simulink library "CampusEnergyModeling"  (Simulink 8.1)
settings: Solver=ode45  StartTime=0.0  StopTime=10.0  RelTol=1e-3
values from neighbouring files (symbols this model uses):
  a = alpha    [GenericInverter_cb.m]
  b = beta    [GenericInverter_cb.m]
  c = gamma    [GenericInverter_cb.m]
  look_Pin = lookup_out ./ lookup_eff    [GenericInverter_cb.m]
  look_Pout = lookup_out    [GenericInverter_cb.m]
undefined symbols (not defined in the file or in its folder): j, magnitude
libraries: powerlib x5, simulink x3
settings Model: Creator=sfrank1  LastModifiedBy=sfrank1

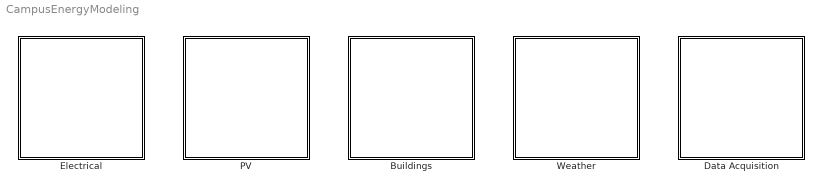
== system CampusEnergyModeling ==
  Buildings : Subsystem  Tag=Weather  Description=Contains blocks for acquiring and manipulating weather data.
      mask Display: disp('Buildings')
  Data Acquisition : Subsystem  Tag=Weather  Description=Contains blocks for acquiring and manipulating weather data.
      mask Display: disp('Data\nAcquisition')
  Electrical : Subsystem  Tag=Weather  Description=Contains blocks for acquiring and manipulating weather data.
      mask Display: disp('Electrical')
  PV : Subsystem  Tag=Weather  Description=Contains blocks for acquiring and manipulating weather data.
      mask Display: disp('PV')
  Weather : Subsystem  Tag=Weather  Description=Contains blocks for acquiring and manipulating weather data.
      mask Display: disp('Weather')

== system CampusEnergyModeling/Buildings ==
  E+ Building : M-S-Function  FunctionName=mlepSimulinkBlk  Parameters=progname, modelfile, weatherfile, workdir, timeout, port, host, bcvtbdir, deltaT, noutputd  mask(EnergyPlus Cosimulation){progname='C:\EnergyPlusV8-0-0\RunEPlus.bat', modelfile='\path\to\dir\idf_file', weatherfile='USA_IL_Chicago-OHare.Intl.AP.725300_TMY3', workdir='\path\to\dir', timeout=80000, port=0, host='', bcvtbdir='', deltaT=900, noutputd=2}
      mask prompts: progname "E+ Executable Path"; modelfile "IDF File (without extension)"; weatherfile "Weather Profile"; workdir "Working Directory"; timeout "Timeout (in milliseconds)"; port "Socket Port (0 = any available)"; host "Socket Host ('' = local host)"; bcvtbdir "BCVTB Directory"; deltaT "Time Step (in seconds)"; noutputd "Number of Real Outputs"
      mask help: This block implements cosimulation with EnergyPlus by allowing Simulink to exchange input and output data with it. Currently, EnergyPlus only supports real data.
      mask Help:
      | This block implements cosimulation with EnergyPlus by allowing Simulink to exchange input and output data with it.
      | 
      | When a simulation starts, EnergyPlus is also started. It will then run in parallel with Simulink. They exchange input and output data via socket communication. When the simulation terminates, EnergyPlus will exit.
      | 
      | Refer to the manuals of MLE+ and/or BCVTB/EnergyPlus for details.
      | 
      | INPUTS:
      | - real: real vector input to EnergyPlus.
      | 
      | OUTPUTS:
      | - flag: status of EnergyPlus (0 if OK, if flag is non-zero, the simulation should stop).
      | - time: current simulation time of EnergyPlus, in seconds.
      | - real: real vector output from EnergyPlus.
      mask Display:
      | image(imread('building.png'))
      | disp('E+\nCosimulation');
      | 
      | % Inputs
      | port_label('input', 1, 'real');
      | 
      | % Outputs
      | port_label('output', 1, 'flag');
      | port_label('output', 2, 'time');
      | port_label('output', 3, 'real');
  E+ Plant : M-S-Function  FunctionName=mlepSimulinkBlk  Parameters=progname, modelfile, weatherfile, workdir, timeout, port, host, bcvtbdir, deltaT, noutputd  mask(EnergyPlus Cosimulation){progname='C:\EnergyPlusV8-0-0\RunEPlus.bat', modelfile='\path\to\dir\idf_file', weatherfile='USA_IL_Chicago-OHare.Intl.AP.725300_TMY3', workdir='\path\to\dir', timeout=80000, port=0, host='', bcvtbdir='', deltaT=900, noutputd=2}
      mask prompts: progname "E+ Executable Path"; modelfile "IDF File (without extension)"; weatherfile "Weather Profile"; workdir "Working Directory"; timeout "Timeout (in milliseconds)"; port "Socket Port (0 = any available)"; host "Socket Host ('' = local host)"; bcvtbdir "BCVTB Directory"; deltaT "Time Step (in seconds)"; noutputd "Number of Real Outputs"
      mask help: This block implements cosimulation with EnergyPlus by allowing Simulink to exchange input and output data with it. Currently, EnergyPlus only supports real data.
      mask Help:
      | This block implements cosimulation with EnergyPlus by allowing Simulink to exchange input and output data with it.
      | 
      | When a simulation starts, EnergyPlus is also started. It will then run in parallel with Simulink. They exchange input and output data via socket communication. When the simulation terminates, EnergyPlus will exit.
      | 
      | Refer to the manuals of MLE+ and/or BCVTB/EnergyPlus for details.
      | 
      | INPUTS:
      | - real: real vector input to EnergyPlus.
      | 
      | OUTPUTS:
      | - flag: status of EnergyPlus (0 if OK, if flag is non-zero, the simulation should stop).
      | - time: current simulation time of EnergyPlus, in seconds.
      | - real: real vector output from EnergyPlus.
      mask Display:
      | image(imread('chiller_plant.jpg'))
      | disp('E+\nCosimulation');
      | 
      | % Inputs
      | port_label('input', 1, 'real');
      | 
      | % Outputs
      | port_label('output', 1, 'flag');
      | port_label('output', 2, 'time');
      | port_label('output', 3, 'real');

== system CampusEnergyModeling/Data Acquisition ==

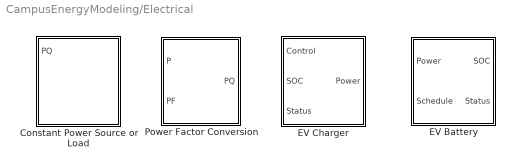
== system CampusEnergyModeling/Electrical ==
  Constant Power Source or Load : Subsystem  mask(Constant Power Source/Load){Conven=source, PNom=5000, QNom=2000, VNom=480, fNom=60, VLow=0.7}
      mask prompts: Conven "Electrical convention"; PNom "Nominal three-phase real power (W)"; QNom "Nominal three-phase reactive power (VAR)"; VNom "Nominal line-to-line voltage (VRMS)"; fNom "Nominal frequency (Hz)"; VLow "Lower voltage limit (pu)"
      mask help: Implements a controllable three-phase, constant power source or load, where VI* = P + jQ (in per-unit).
      mask init:
      | % Call initialization to calculate block variables
      | InputGain = ...
      |     ConstantPowerSourceLoad_cb(gcb, 'init', ...
      |     Conven, PNom, QNom, VNom, fNom, VLow);
      mask Help:
      | Implements a controllable three-phase, constant power source or load in SimPowerSystems (phasor mode). The load characteristic is given by P + jQ = sqrt(3)VI*, in which
      |     V = Positive sequence line-to-line voltage (V)
      |     I = Positive sequence phase current (A)
      |     P = Positive sequence real power (from PQ input)
      |     Q = Positive sequence reactive power (from PQ input)
      | 
      | The block supplies P + jQ if the source convention is specified and consumes P + jQ if the load convention is specified.
      | 
      | The nominal input fields in the mask are used to initialize the block parameters. If the nominal values are close to the actual values during simulation, then the block will converge more rapidly.
      | 
      | If the positive sequence voltage falls below the per-unit lower voltage limit (on the base specified by the nominal line-to-line voltage), then the block will behave as a constant current source rather than a constant power source, with the current magnitude capped at the level required to supply full power at V = 0.7 pu. This feature avoids current runaway that would otherwise occur during voltage collapes.
      | 
      | NOTE: This block is compatible only with SimPowerSystems' phasor simulation mode.
      mask TypeOptions Conven: source | load
  EV Battery : Subsystem  mask(Electric Vehicle Battery){capacity=24000, initSOC=0.3}
      mask prompts: capacity "Battery capacity (Wh)"; initSOC "Initial state of charge (fraction)"
      mask help: Implements a simple, lossless model for an electric vehicle (EV) battery.
      mask Help:
      | Implements a simple, lossless model for an electric vehicle (EV) battery.
      | 
      | The block accepts the following inputs:
      | •	Power = The charging power for the battery (W)
      | •	Schedule = 1 if the EV is connected to the charging station, 0 otherwise
      | 
      | The block outputs two signals:
      | •	SOC = The battery state of charge (fraction)
      | •	Status = EV status: -1 for not present, 0 for present and accepting charge, 1 for present but battery full
      | 
      | Internally, the battery is modeled using a simple integrator for the input power, capped at 100% SOC. Battery SOC resets to the specified initial value whenever the EV first connects to the charging station. The battery is lossless.
  EV Charger : Subsystem  mask(Electric Vehicle Charging Station){rating=6240, capacity=24000, maxresponse=1000, ramp=1000}
      mask prompts: rating "Charger rating (W)"; capacity "Connected EV battery capacity (Wh)"; maxresponse "Desired +/- regulatory response capability (W)"; ramp "Maximum ramp rate (W/s)"
      mask help: Implements a simple model for an electric vehicle charging station. Accepts connections for the EV state of charge and status as well as an external control signal requesting a regulatory deviation from the current charging setpoint. Outputs a charging power.
      mask Help:
      | Implements a simple model for an electric vehicle (EV) charging station.
      | 
      | The block accepts the following inputs:
      | •	Control = Signal requesting regulatory control of power consumed (+/- deviation from setpoint) (W)
      | •	SOC = EV battery state of charge (fraction)
      | •	Status = EV status: -1 for not present, 0 for present and accepting charge, 1 for present but battery full
      | 
      | The block outputs the charging power to the EV battery.
      | 
      | The charger uses a preset charging power profile based on the EV battery state of charge (SOC). As the SOC approaches 100%, the charger tapers the charge rate to zero. In addition, the charger monitors the connection status of the EV and sets charging power to zero if the EV is disconnected or has a full battery.
      | 
      | The 'Control' signal requests regulatory control of the EV charging load as a deviation from the current charging setpoint. This allows the EV charger to participate in demand response or regulation of distributed generation (such as smoothing output from a photovoltaic array). The charger attempts to maintain the active response capability specified in the block mask by operating at less than maximum charging capacity. It can then respond to the control signal within its present charging limits.
      | 
      | For example, if, given the current battery SOC, the charging profile for the EV battery specifies 5000 W and the requested regulatory response capability is +/- 1000 W, then the EV charger will charge at a setpoint of 4000 W +/- the requested control action, within the limits of the charger. If the requested control action is -500 W, then the EV charger will reduce output to 4000 - 500 = 3500 W.
      | 
      | The ability of the charger to respond to the control action is limited by several factors:
      | 1.	The output cannot exceed either its specified rating or the maximum charge rate given by the battery charging profile.
      | 2.	The output cannot be less than zero.
      | 3.	The output cannot change at a rate greater than the specified maximum ramp rate (W/s).
  Power Factor Conversion : Subsystem  mask(Power Factor Conversion){pfType=Lagging}
      mask prompts: pfType "Type of power factor"
      mask help: Converts a real input power and power factor to a vector of real and reactive power.
      mask init:
      | % Set multiplier for Q based on load type
      | if pfType == 1
      |     % Leading
      |     leadlag = -1;
      | else
      |     % Lagging
      |     leadlag = 1;
      | end
      mask Help: Converts a real input power and power factor to a vector of real and reactive power. The output is a vector [P Q] computed from the input power P, input power factor PF, and whether the signal indicates leading or lagging power (selectable in the block mask).
      mask TypeOptions pfType: Leading | Lagging

== system CampusEnergyModeling/PV ==
  Generic Inverter : Subsystem  mask(Generic Inverter){model_type=Fixed Efficiency, fixed_eff=0.95, alpha=1, beta=0.01, gamma=0.001, lookup_pair=Input Power + Output Power, lookup_in=[0, 10, 25, 50, 75, 100], lookup_out=[0, 9, 24, 49, 73, 97], lookup_eff=[0.10, 0.80, 0.87, 0.93, 0.90, 0.88]}
      mask prompts: model_type "Inverter model"; fixed_eff "Efficiency"; alpha "Constant loss coefficient (W)"; beta "Linear loss coefficient (W/W)"; gamma "Quadratic loss coefficient (W/W²)"; lookup_pair "Specify..."; lookup_in "Input power (W)"; lookup_out "Output power (W)"; lookup_eff "Efficiency"
      mask help:
      | Implements the efficiency characteristic for a generic PV inverter using one of three models:
      | - Fixed efficiency
      | - Quadratic loss model
      | - Lookup table
      |
      | See the help for details for each of these models.
      mask init:
      | % Call initialization to calculate block variables
      | [a, b, c, look_Pin, look_Pout] = ...
      |     GenericInverter_cb(gcb, 'init', model_type, ...
      | 	fixed_eff, alpha, beta, gamma, ...
      |     lookup_pair, lookup_in, lookup_out, lookup_eff);
      mask Help:
      | This block implements the efficiency characteristic for a generic PV inverter using one of three models:
      | - Fixed efficiency
      | - Quadratic loss model
      | - Lookup table
      | 
      | Fixed Efficiency:
      | Specify the fixed inverter efficiency as a fraction.
      | 
      | Quadratic Loss Model:
      | Specify the loss model coefficients such that
      | Pout = Pin - (alpha + beta*Pin + gamma*Pin²).
      | 
      | Lookup Table:
      | Specify two of the following three vectors: input power, output power, and efficiency. Efficiencies must be entered as fractions and vector lengths must match. The block automatically calculates the appropriate input-output power characteristic from the inputs provided according to the relationship Efficiency = Pout / Pin.
      | 
      | CAUTION: When using the lookup table, do not include zeros in the efficiency vector. Otherwise, a divide by zero error may result.
      mask TypeOptions model_type: Fixed Efficiency | Quadratic | Lookup Table
      mask Callback model_type:
      | % Dynamic mask callback
      | GenericInverter_cb(gcb, 'model_type')
      mask TypeOptions lookup_pair: Input Power + Output Power | Input Power + Efficiency | Output Power + Efficiency
      mask Callback lookup_pair:
      | % Dynamic mask callback
      | GenericInverter_cb(gcb, 'lookup_pair')
  PV Smoothing : TransferFcn  Denominator=[tau 1]  mask(Photovoltaic Array Smoothing){sel=Array Size and Power Density, tc=15, area=33000, size=1e6, density=150, coverage=0.2}
      mask prompts: sel "Specify..."; tc "Time constant (s)"; area "Array area (m²)"; size "Array size (W)"; density "Panel nominal power density (W/m²)"; coverage "Panel ground coverage ratio (fraction)"
      mask help: Implements a low pass filter to model the smoothing effect of a utility-scale PV array.
      mask init:
      | % Call initialization to calculate block variables
      | tau = PVSmoothing_cb(gcb, 'init', ...
      |     sel, tc, area, size, density, coverage);
      mask Help:
      | This block implements a low pass filter to model the smoothing effect of a utility-scale PV array per the empirical model presented in Marcos et al. (2011) (see References). The smoothing is done by a unity-gain low pass filter with transfer function
      | 
      | Output / Input = 1 / (tau*s + 1)
      | 
      | in which time constant tau may either be defined directly or estimated from the array area. The empirical formula of Marcos et al. estimates tau as
      | 
      | tau = sqrt(A) / (2*pi*0.020)
      | 
      | in which A is the physical array area in hectares (1 Ha = 10000 m²). Array area A may be specified directly or calculated from the array size, panel power density, and ground coverage ratio (defined as the fraction of ground area occupied by the actual PV panels).
      | 
      | Notes:
      | 1. This block includes a continuous time low pass filter. Use caution when attempting to use this block within models with fixed time larger than the smoothing time constant; the Simulink solver may generate an error.
      | 
      | References:
      | J. Marcos et al., "From irradiance to output power fluctuations: the PV plant as a low pass filter", Progress In Photovoltaics: Research And Applications, 2011, 19, 505-510.
      mask TypeOptions sel: Time Constant | Array Area | Array Size and Power Density
      mask Callback sel: PVSmoothing_cb(gcb, 'dynamic_mask')
      mask Display: plot([1 2 3],[1 1 0])
  PVWatts Cosimulation : M-S-Function  FunctionName=pvwatts_sfun  Parameters=lat, lon, start_time, tz, time_step, system_size, derate, azimuth, tilt, track_mode, rotlim, t_ref, t_noct, gamma, i_ref, poa_cutin, init_tcell, init_poa, output_dc, output_celltemp, output_poa  mask(PVWatts Cosimulation){lat=39.74, lon=-105.18, start_time=2012-01-01 00:00:00, tz=-6, time_step=600, system_size=1000, derate=0.95, azimuth=180, tilt=39.74, use_lat_tilt=on, track_mode=Fixed, rotlim=45, use_cell_data=off, t_ref=25, t_noct=45, gamma=-0.5, i_ref=1000, poa_cutin=0, init_tcell=25, init_poa=0, output_dc=on, output_celltemp=on, output_poa=on}
      mask prompts: lat "Latitude"; lon "Longitude"; start_time "Initial date/time (yyyy-mm-dd HH:MM:SS)"; tz "Time zone (offset from UTC)"; time_step "Time step (s)"; system_size "Array nameplate capacity (W)"; derate "System derate factor (0-1)"; azimuth "Azimuth angle (N = 0°, E = 90°, S = 180°, W = 270°)"; tilt "Tilt angle"; use_lat_tilt "Use latitude tilt"; track_mode "Tracking mode"; rotlim "Tracker rotation limit (+/-)"; use_cell_data "Customize photovoltaic cell data"; t_ref "Reference cell temperature (°C)"; t_noct "Nominal operating cell temperature (°C)"; gamma "Maximum power temperature coefficient (%/°C)"; i_ref "Irradiance condition for cell rating (W/m²)"; poa_cutin "Minimum irradiance for operation (W/m²)"; init_tcell "Initial cell temperature (°C)"; init_poa "Initial plane of array irradiance (W/m²)"; output_dc "Output DC power (W)"; output_celltemp "Output cell temperature (°C)"; output_poa "Output plane of array irradiance (W/m²)"
      mask help:
      | This block implements cosimulation of a photovoltaic (PV) array using the PVWatts module of the SAM Simulation Code (SSC) SDK. Data entry is organized in four tabs:
      | 1. Time and Location: where the array is located and when the simulation occurs.
      | 2. Array: PV array nameplate rating and physical characteristics.
      | 3. Cell: Customized model parameters for the PV cells (optional).
      | 4. Simulation: Initial conditions and simulation options.
      |
      | See the block help for more information.
      mask init:
      | PVWatts_cb(gcb, 'redraw_mask');
      mask Help:
      | This block implements cosimulation of a photovoltaic (PV) array using the PVWatts (pvwattsfunc) module of the SAM Simulation Code (SSC) SDK. The cosimulation runs in SSC at the time step specified in the 'Time and Location' tab (which need not be identical to the Simulink time step).
      | 
      | The block inputs accept weather data synced to the simulation time stamp:
      | 1. Beam irradiance (W/m²) - Also known as "direct normal irradiance"
      | 2. Diffuse irradiance (W/m²) - Also known as "diffuse horizontal irradiance"
      | 3. Ambient temperature (°C)
      | 4. Wind speed (m/s)
      | 
      | The block mask provides inputs for most (although not all) of the remaining PV array model parameters available for PVWatts in SSC, such as the array ratings, physical location and orientation, PV cell characteristics, etc. The four input tabs in the block mask are:
      | 1. Time and Location: where the array is located and when the simulation occurs.
      | 2. Array: PV array nameplate rating and physical characteristics.
      | 3. Cell: Customized model parameters for the PV cells (optional).
      | 4. Simulation: Initial conditions and simulation options.
      | 
      | The block outputs are, in order:
      | 1. Array DC output power (W)
      | 2. Array cell temperature (°C)
      | 3. Plane of array irradiance (W/m²)
      | Each output may be individually enabled or disabled on the 'Simulation' tab. Please note that enabling or disabling outputs will change the number of output ports on the block, possibly disrupting existing signal connections in Simulink.
      | 
      | Notes:
      | 1. CAUTION: Checking 'Use latitude tile' will discard the existing tilt angle and replace it with the absolute value of the latitude.
      | 2. CAUTION: Unchecking 'Customize photovoltaic cell data' will discard any existing customizations in the PV cell data fields.
      | 3. The block is designed to model the DC operation of a PV array only. Therefore, no inverter efficiency mask parameter or AC power output are provided. To model inverter losses, apply an external inverter model to the DC power output, such as the 'Generic Inverter' model available in the Campus Modeling Simulink library.
      | 
      | 
      | Detailed documentation for the SSC SDK is available for download at:
      | https://sam.nrel.gov/content/sam-simulation-core-sdk
      | Additional description for the SSC module input and output variables may be obtained using the SSCdev application distributed with SSC SDK; see the SSC SDK documentation for usage instructions.
      mask Callback lat: PVWatts_cb(gcb, 'use_lat_tilt');
      mask Callback use_lat_tilt: PVWatts_cb(gcb, 'use_lat_tilt');
      mask TypeOptions track_mode: Fixed | 1-Axis | 2-Axis | Azimuth Axis
      mask Callback track_mode: PVWatts_cb(gcb, 'track_mode');
      mask Callback use_cell_data: PVWatts_cb(gcb, 'use_cell_data');
      mask Display:
      | % This mask display is automatically generated by PVWatts_cb()
      | image('pvwatts_light.png')
      | disp('PVWatts\nCosimulation')
      | 
      | % Label input ports
      | port_label('input', 1, 'Beam'); % Beam irradiance (W/m^2)
      | port_label('input', 2, 'Diffuse'); % Diffuse irradiance (W/m^2)
      | port_label('input', 3, 'Temp'); % Ambient temperature (deg C)
      | port_label('input', 4, 'Wind'); % Wind speed (m/s)
      | 
      | % Label output ports
      | port_label('output', 1, 'DC power'); % DC output power (W)
      | port_label('output', 2, 'Cell Temp'); % Cell Temperature (deg C)
      | port_label('output', 3, 'POA Irradiance'); % % Point of array irradiance

== system CampusEnergyModeling/Weather ==
  Weather Data : Subsystem  mask(Weather Data From File){fname=TMY3.mat, initbus=off}
      mask prompts: fname "Weather file"; initbus "Create Simulink bus definition automatically?"
      mask help:
      | Reads weather data from the specified binary file and outputs it as a Simulink bus signal.
      |
      | The utility function convertTMY3() to creates a .MAT file compatible with this block. Use of this block requires that a Simulink bus object named 'BusDef_Weather' be defined in the base workspace. See the block help for details.
      mask init:
      | % Run initialization callback
      | Weather_cb(gcb, 'init', fname, initbus)
      mask Help:
      | This block reads weather data from a binary (.MAT) file and outputs it as a Simulink bus signal. Because the block uses Simulink's 'From File' block internally for file I/O, there are several requirements for it to function correctly:
      | 1. The user must create a bus definition named 'BusDef_Weather' for the weather data and save it to the base MATLAB workspace. This bus definition will be automatically generated from the weather file if the 'Create Simulink bus definition automatically' checkbox is checked.
      | 2. The .MAT file must contain time series objects organized within a structure (struct) object called 'ans'.
      | 3. The structure must match the bus definition. (If the block is allowed to automatically generate the Simulink bus definition, this requirement will be satisfied.)
      | 3. The .MAT file must be version 7.3 or higher.
      | 4. All time series in the .MAT file must have units of seconds; otherwise Simulink will interpret them incorrectly.
      | 
      | The utility script convertTMY3() is available to convert TMY3-formatted weather data into MATLAB time series objects compatible with these requirements. See the convertTMY3() function documentation for details.
      mask Display:
      | image(imread('SkyImage.png'))
      | port_label('output', 1, 'data');

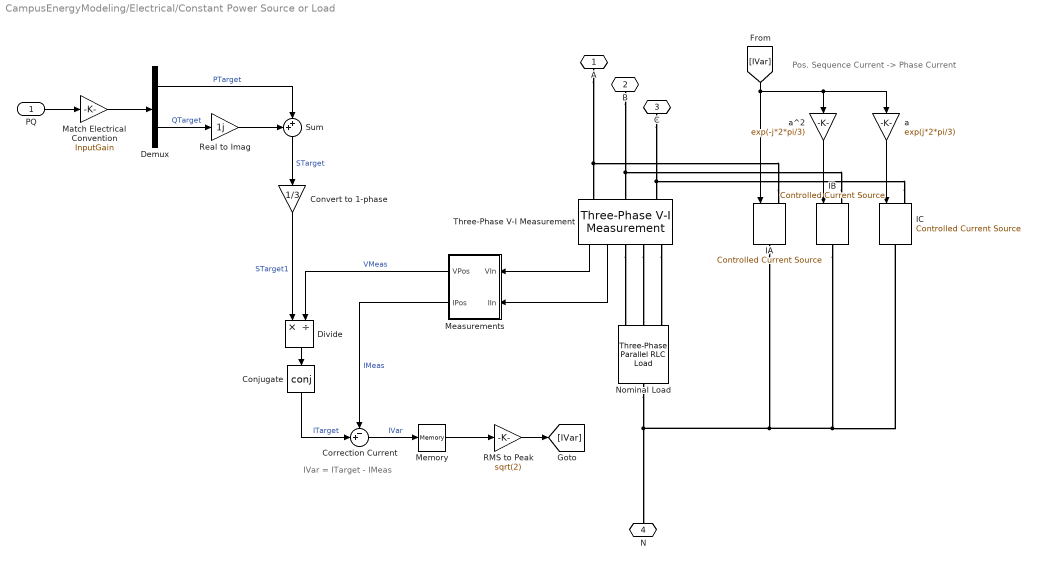
== system CampusEnergyModeling/Electrical/Constant Power Source or Load ==
  note: Pos. Sequence Current -> Phase Current
  note: IVar = ITarget - IMeas
  PQ : Inport  PortDimensions=2
  Conjugate : Math  Operator=conj  SaturateOnIntegerOverflow=on
  Convert to 1-phase : Gain  Gain=1/3
  Correction Current : Sum  Inputs=-+|
  Demux : Demux  Outputs=2
  Divide : Product  Inputs=*/
  IA : powerlib/Electrical Sources/Controlled Current Source  Initialize=off  Source_Type=AC  Amplitude=0  Phase=0  Frequency=0  Measurements=Current
  IB : powerlib/Electrical Sources/Controlled Current Source  Initialize=off  Source_Type=AC  Amplitude=0  Phase=0  Frequency=0  Measurements=Current
  IC : powerlib/Electrical Sources/Controlled Current Source  Initialize=off  Source_Type=AC  Amplitude=0  Phase=0  Frequency=0  Measurements=Current
  Match Electrical Convention : Gain  Gain=InputGain
  Measurements : Subsystem
  Memory : Memory
  Nominal Load : powerlib/Elements/Three-Phase Parallel RLC Load  LConnTagsString=A|B|C  RConnTagsString=N  Configuration=Y (neutral)  NominalVoltage=VNom  NominalFrequency=fNom  ActivePower=max(PNom*InputGain,1e-3)  InductivePower=max(QNom*InputGain,0)  CapacitivePower=max(-QNom*InputGain,0)  Measurements=None  LoadType=constant PQ
  RMS to Peak : Gain  Gain=sqrt(2)
  Real to Imag : Gain  Gain=1j
  Sum : Sum  Inputs=++|
  Three-Phase V-I Measurement : powerlib/Measurements/Three-Phase V-I Measurement  VoltageMeasurement=phase-to-ground  SetLabelV=off  LabelV=Vabc  Vpu=off  VpuLL=off  CurrentMeasurement=yes  SetLabelI=off  LabelI=Iabc  Ipu=off  Pbase=100e6  Vbase=VNom  OutputType=Complex  PhasorSimulation=on  PSBequivalent=0
  a : Gain  Gain=exp(j*2*pi/3)
  a^2 : Gain  Gain=exp(-j*2*pi/3)
  A : PMIOPort  Port=1  Side=Left
  B : PMIOPort  Port=2  Side=Left
  C : PMIOPort  Port=3  Side=Left
  N : PMIOPort  Port=4  Side=Left
  wires:
  Measurements/2(IPos) -> Correction Current/1  "IMeas"
  Measurements/1(VPos) -> Divide/2  "VMeas"
  Demux/1 -> Sum/2  "PTarget"
  Real to Imag/1 -> Sum/1
  Match Electrical Convention/1 -> Demux/1
  PQ/1 -> Match Electrical Convention/1
  Memory/1 -> RMS to Peak/1
  RMS to Peak/1 -> [IVar]
  Conjugate/1 -> Correction Current/2  "ITarget"
  Correction Current/1 -> Memory/1  "IVar"
  a/1 -> IC/1
  a^2/1 -> IB/1
  [IVar] -> a/1, a^2/1, IA/1
  Divide/1 -> Conjugate/1
  Convert to 1-phase/1 -> Divide/1  "STarget1"
  Sum/1 -> Convert to 1-phase/1  "STarget"
  Demux/2 -> Real to Imag/1  "QTarget"
  Three-Phase V-I Measurement/2 -> Measurements/2(IIn)
  Three-Phase V-I Measurement/1 -> Measurements/1(VIn)
  connections:
  IC/RConn1 -- N/RConn1 -- Nominal Load/RConn1 -- IA/RConn1 -- IB/RConn1
  Three-Phase V-I Measurement/RConn3 -- Nominal Load/LConn3
  Three-Phase V-I Measurement/RConn2 -- Nominal Load/LConn2
  Three-Phase V-I Measurement/RConn1 -- Nominal Load/LConn1
  IC/LConn1 -- Three-Phase V-I Measurement/LConn3 -- C/RConn1
  IB/LConn1 -- Three-Phase V-I Measurement/LConn2 -- B/RConn1
  IA/LConn1 -- Three-Phase V-I Measurement/LConn1 -- A/RConn1

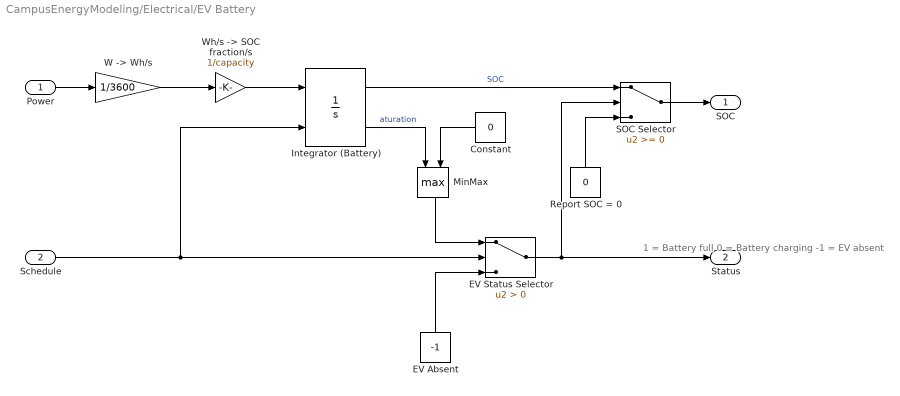
== system CampusEnergyModeling/Electrical/EV Battery ==
  note: 1 = Battery full
      | 0 = Battery charging
      | -1 = EV absent
  Power : Inport
  Schedule : Inport  Port=2
  Constant : Constant  Value=0
  EV Absent : Constant  Value=-1
  EV Status Selector : Switch  Criteria=u2 > Threshold
  Integrator (Battery) : Integrator  ExternalReset=rising  InitialCondition=initSOC  LimitOutput=on  UpperSaturationLimit=1  LowerSaturationLimit=0  ShowSaturationPort=on  ContinuousStateAttributes='SOC'
  MinMax : MinMax  Function=max  Inputs=2
  Report SOC = 0 : Constant  Value=0
  SOC Selector : Switch
  "W -> Wh/s" : Gain  Gain=1/3600
  "Wh/s -> SOC fraction/s" : Gain  Gain=1/capacity
  SOC : Outport
  Status : Outport  Port=2
  wires:
  "W -> Wh/s"/1 -> "Wh/s -> SOC fraction/s"/1
  Power/1 -> "W -> Wh/s"/1
  "Wh/s -> SOC fraction/s"/1 -> Integrator (Battery)/1
  Schedule/1 -> EV Status Selector/2, Integrator (Battery)/2
  EV Absent/1 -> EV Status Selector/3
  EV Status Selector/1 -> SOC Selector/2, Status/1
  Integrator (Battery)/2 -> MinMax/1  "aturation"
  MinMax/1 -> EV Status Selector/1
  Constant/1 -> MinMax/2
  Integrator (Battery)/1 -> SOC Selector/1  "SOC"
  SOC Selector/1 -> SOC/1
  Report SOC = 0/1 -> SOC Selector/3

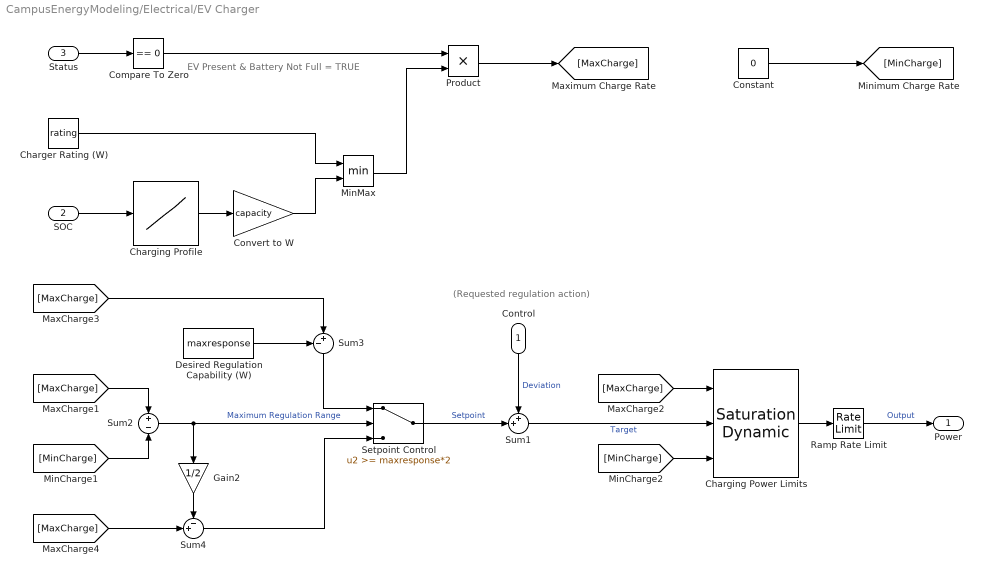
== system CampusEnergyModeling/Electrical/EV Charger ==
  note: EV Present & Battery Not Full = TRUE
  note: (Requested regulation action)
  Control : Inport
  SOC : Inport  Port=2
  Status : Inport  Port=3
  Charger Rating (W) : Constant  Value=rating
  Charging Power Limits : simulink/Discontinuities/Saturation Dynamic  OutMin=[]  OutMax=[]  OutDataTypeStr=Inherit: Same as second input  OutDataType=fixdt(1, 16)  OutScaling=2^-10  DoSatur=off
  Charging Profile : Lookup_n-D  NumberOfTableDimensions=1  BreakpointsForDimension1=[0.00 0.10 0.20 0.80 0.99 1.00]  IndexSearchMethod=Linear search  BeginIndexSearchUsingPreviousIndexResult=on  Table=[0.10 0.20 1.00 1.00 0.02 0.00]  ExtrapMethod=Clip  UseLastTableValue=on  RndMeth=Simplest  InputSameDT=on
  Compare To Zero : simulink/Logic and Bit Operations/Compare To Zero  relop===  OutDataTypeStr=boolean
  Constant : Constant  Value=0
  Convert to W : Gain  Gain=capacity
  Desired Regulation Capability (W) : Constant  Value=maxresponse
  Gain2 : Gain  Gain=1/2
  MinMax : MinMax  Inputs=2
  Product : Product
  Ramp Rate Limit : RateLimiter  RisingSlewLimit=ramp  FallingSlewLimit=-ramp  SampleTimeMode=inherited
  Setpoint Control : Switch  Threshold=maxresponse*2
  Sum1 : Sum  Inputs=++|
  Sum2 : Sum  Inputs=+-
  Sum3 : Sum  Inputs=-+|
  Sum4 : Sum  Inputs=-+|
  Power : Outport
  wires:
  Sum1/1 -> Charging Power Limits/2  "Target"
  Ramp Rate Limit/1 -> Power/1  "Output"
  SOC/1 -> Charging Profile/1
  Charging Profile/1 -> Convert to W/1
  Charging Power Limits/1 -> Ramp Rate Limit/1
  Status/1 -> Compare To Zero/1
  Compare To Zero/1 -> Product/1
  Convert to W/1 -> MinMax/2
  Charger Rating (W)/1 -> MinMax/1
  MinMax/1 -> Product/2
  Product/1 -> [MaxCharge]
  Constant/1 -> [MinCharge]
  Control/1 -> Sum1/1  "Deviation"
  [MaxCharge] -> Charging Power Limits/1
  [MinCharge] -> Charging Power Limits/3
  Sum2/1 -> Gain2/1, Setpoint Control/2  "Maximum Regulation Range"
  [MaxCharge] -> Sum2/1
  [MinCharge] -> Sum2/2
  Setpoint Control/1 -> Sum1/2  "Setpoint"
  Sum3/1 -> Setpoint Control/1
  [MaxCharge] -> Sum4/2
  Gain2/1 -> Sum4/1
  Sum4/1 -> Setpoint Control/3
  [MaxCharge] -> Sum3/2
  Desired Regulation Capability (W)/1 -> Sum3/1

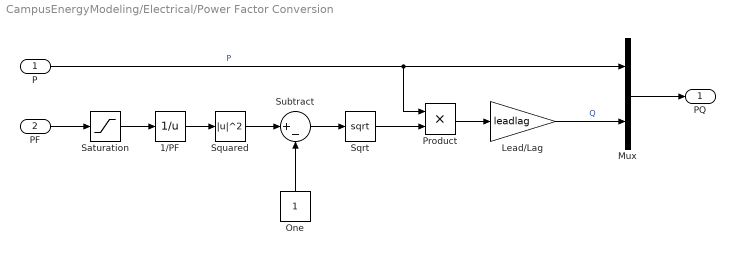
== system CampusEnergyModeling/Electrical/Power Factor Conversion ==
  P : Inport
  PF : Inport  Port=2
  1/PF : Math  Operator=reciprocal  SaturateOnIntegerOverflow=on
  Lead/Lag : Gain  Gain=leadlag
  Mux : Mux  Inputs=2
  One : Constant
  Product : Product
  Saturation : Saturate  UpperLimit=1  LowerLimit=0  ZeroCross=off
  Sqrt : Sqrt  SaturateOnIntegerOverflow=on
  Squared : Math  Operator=magnitude^2  SaturateOnIntegerOverflow=on
  Subtract : Sum  Inputs=|+-
  PQ : Outport
  wires:
  Subtract/1 -> Sqrt/1
  Sqrt/1 -> Product/2
  Mux/1 -> PQ/1
  Product/1 -> Lead/Lag/1
  PF/1 -> Saturation/1
  1/PF/1 -> Squared/1
  One/1 -> Subtract/2
  Squared/1 -> Subtract/1
  P/1 -> Product/1, Mux/1  "P"
  Lead/Lag/1 -> Mux/2  "Q"
  Saturation/1 -> 1/PF/1

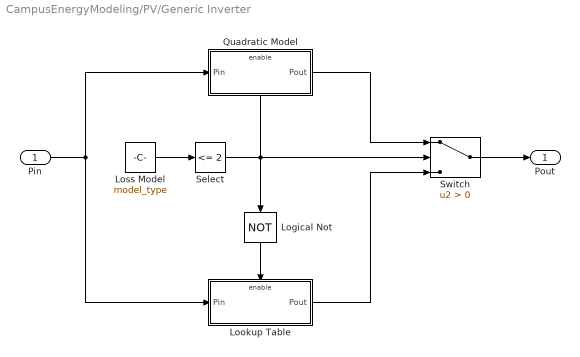
== system CampusEnergyModeling/PV/Generic Inverter ==
  Pin : Inport
  Logical Not : Logic  Operator=NOT  IconShape=distinctive  AllPortsSameDT=off  OutDataTypeStr=boolean
  Lookup Table : Subsystem  TreatAsAtomicUnit=on
  Loss Model : Constant  Value=model_type
  Quadratic Model : Subsystem  TreatAsAtomicUnit=on
  Select : simulink/Logic and Bit Operations/Compare To Constant  relop=<=  const=2  OutDataTypeStr=boolean
  Switch : Switch  Criteria=u2 > Threshold  ZeroCross=off
  Pout : Outport
  wires:
  Switch/1 -> Pout/1
  Loss Model/1 -> Select/1
  Logical Not/1 -> Lookup Table/Enable
  Pin/1 -> Quadratic Model/1(Pin), Lookup Table/1(Pin)
  Quadratic Model/1(Pout) -> Switch/1
  Select/1 -> Logical Not/1, Switch/2, Quadratic Model/Enable
  Lookup Table/1(Pout) -> Switch/3

== system CampusEnergyModeling/Weather/Weather Data ==
  From File : FromFile  FileName=TMY3.mat  OutDataTypeStr=Bus: BusDef_Weather  SampleTime=0  ExtrapolationBeforeFirstDataPoint=Hold first value  ExtrapolationAfterLastDataPoint=Hold last value
  Output : Outport  OutDataTypeStr=Bus: BusDef_Weather
  wires:
  From File/1 -> Output/1

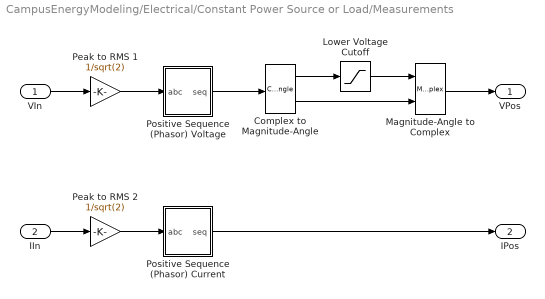
== system CampusEnergyModeling/Electrical/Constant Power Source or Load/Measurements ==
  VIn : Inport
  IIn : Inport  Port=2
  Complex to Magnitude-Angle : ComplexToMagnitudeAngle
  Lower Voltage Cutoff : Saturate  UpperLimit=inf  LowerLimit=VLow*VNom/sqrt(3)
  Magnitude-Angle to Complex : MagnitudeAngleToComplex
  Peak to RMS 1 : Gain  Gain=1/sqrt(2)
  Peak to RMS 2 : Gain  Gain=1/sqrt(2)
  Positive Sequence (Phasor) Current : Subsystem
      mask init:
      | j=sqrt(-1);
      | a=exp(j*2*pi/3);
      | a2=exp(-j*2*pi/3);
  Positive Sequence (Phasor) Voltage : Subsystem
      mask init:
      | j=sqrt(-1);
      | a=exp(j*2*pi/3);
      | a2=exp(-j*2*pi/3);
  VPos : Outport
  IPos : Outport  Port=2
  wires:
  Complex to Magnitude-Angle/2 -> Magnitude-Angle to Complex/2
  Lower Voltage Cutoff/1 -> Magnitude-Angle to Complex/1
  Magnitude-Angle to Complex/1 -> VPos/1
  Complex to Magnitude-Angle/1 -> Lower Voltage Cutoff/1
  Positive Sequence (Phasor) Voltage/1(seq) -> Complex to Magnitude-Angle/1
  Positive Sequence (Phasor) Current/1(seq) -> IPos/1
  Peak to RMS 2/1 -> Positive Sequence (Phasor) Current/1(abc)
  Peak to RMS 1/1 -> Positive Sequence (Phasor) Voltage/1(abc)
  IIn/1 -> Peak to RMS 2/1
  VIn/1 -> Peak to RMS 1/1

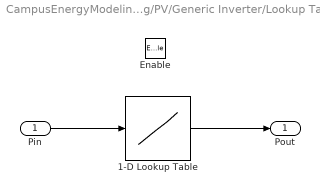
== system CampusEnergyModeling/PV/Generic Inverter/Lookup Table ==
  Pin : Inport
  Enable : EnablePort
  1-D Lookup Table : Lookup_n-D  NumberOfTableDimensions=1  BreakpointsForDimension1=look_Pin  IndexSearchMethod=Linear search  BeginIndexSearchUsingPreviousIndexResult=on  UseOneInputPortForAllInputData=on  Table=look_Pout  RndMeth=Simplest  InputSameDT=on
  Pout : Outport
  wires:
  Pin/1 -> 1-D Lookup Table/1
  1-D Lookup Table/1 -> Pout/1

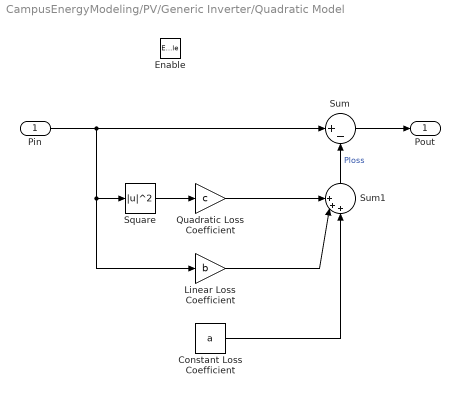
== system CampusEnergyModeling/PV/Generic Inverter/Quadratic Model ==
  Pin : Inport
  Enable : EnablePort
  Constant Loss Coefficient : Constant  Value=a
  Linear Loss Coefficient : Gain  Gain=b
  Quadratic Loss Coefficient : Gain  Gain=c
  Square : Math  Operator=magnitude^2  SaturateOnIntegerOverflow=on
  Sum : Sum  Inputs=|+-
  Sum1 : Sum  Inputs=+++||
  Pout : Outport
  wires:
  Pin/1 -> Sum/1, Linear Loss Coefficient/1, Square/1
  Square/1 -> Quadratic Loss Coefficient/1
  Quadratic Loss Coefficient/1 -> Sum1/1
  Sum/1 -> Pout/1
  Sum1/1 -> Sum/2  "Ploss"
  Linear Loss Coefficient/1 -> Sum1/2
  Constant Loss Coefficient/1 -> Sum1/3

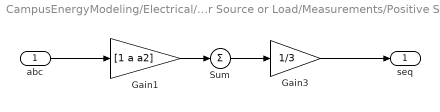
== system CampusEnergyModeling/Electrical/Constant Power Source or Load/Measurements/Positive Sequence (Phasor) Current ==
  abc : Inport
  Gain1 : Gain  Gain=[1 a a2]  SaturateOnIntegerOverflow=on  OutDataTypeStr=Inherit: Same as input  ParamDataTypeStr=Inherit: Same as input
  Gain3 : Gain  Gain=1/3  SaturateOnIntegerOverflow=on  OutDataTypeStr=Inherit: Same as input  ParamDataTypeStr=Inherit: Same as input
  Sum : Sum  Inputs=1  SaturateOnIntegerOverflow=on  InputSameDT=on  OutDataTypeStr=Inherit: Same as first input
  seq : Outport
  wires:
  Sum/1 -> Gain3/1
  Gain1/1 -> Sum/1
  Gain3/1 -> seq/1
  abc/1 -> Gain1/1

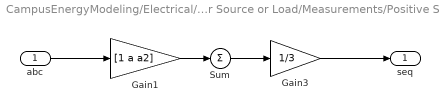
== system CampusEnergyModeling/Electrical/Constant Power Source or Load/Measurements/Positive Sequence (Phasor) Voltage ==
  abc : Inport
  Gain1 : Gain  Gain=[1 a a2]  SaturateOnIntegerOverflow=on  OutDataTypeStr=Inherit: Same as input  ParamDataTypeStr=Inherit: Same as input
  Gain3 : Gain  Gain=1/3  SaturateOnIntegerOverflow=on  OutDataTypeStr=Inherit: Same as input  ParamDataTypeStr=Inherit: Same as input
  Sum : Sum  Inputs=1  SaturateOnIntegerOverflow=on  InputSameDT=on  OutDataTypeStr=Inherit: Same as first input
  seq : Outport
  wires:
  Sum/1 -> Gain3/1
  Gain1/1 -> Sum/1
  Gain3/1 -> seq/1
  abc/1 -> Gain1/1
